simulink subsystem "Simulation_Differential_AGV"  (R2024b)
settings: Solver=VariableStepAuto  StartTime=0.0  StopTime=10.0  RelTol=1e-3
model mask{poseInit=[0 0 0], vInit=[0 0], Ts=0.05, speedLimits=[-2 8]}
  mask prompts: poseInit "Initial position (m,m,rad)"; vInit "Initial speed (m/s, rad/s)"; Ts "Sampling Time (s)"; speedLimits "Speed Limits"
undefined symbols (not defined in the file): DiscIntNeverNeededParam
settings Model: Creator=marti  LastModifiedBy=marti

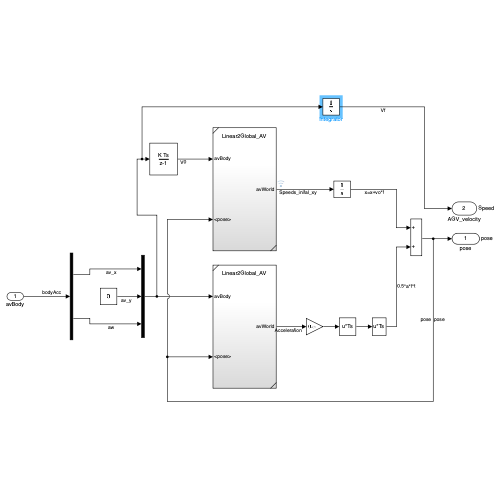
[thumbnail: Simulink's stored preview of the top-level diagram]
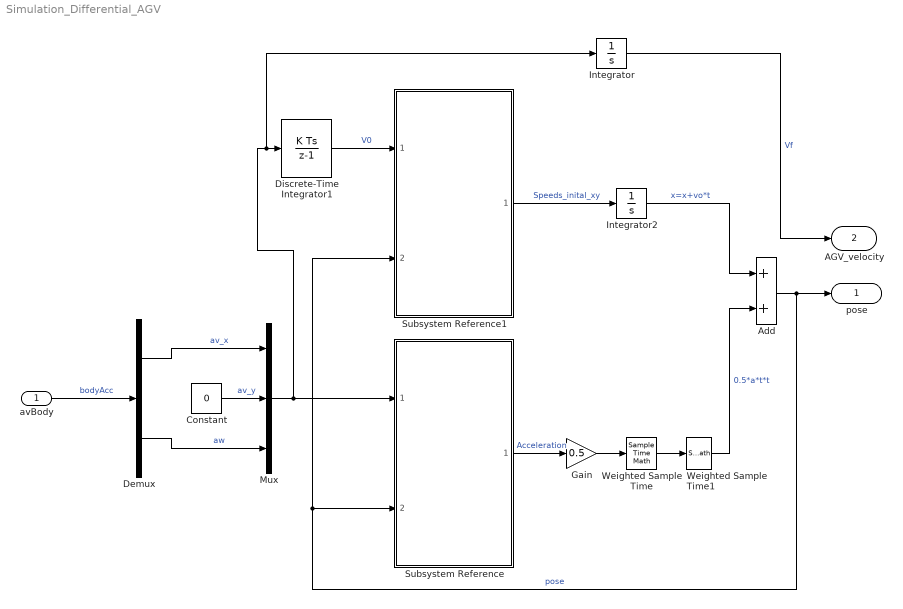
== system Simulation_Differential_AGV ==
  avBody : Inport  PortDimensions=2  SampleTime=Ts
  Add : Sum
  Constant : Constant  Value=0  SampleTime=Ts
  Demux : Demux  Outputs=2
  Discrete-Time Integrator1 : DiscreteIntegrator  InitialCondition=[vInit(1) 0 vInit(2)]  SampleTime=Ts  ICPrevOutput=DiscIntNeverNeededParam  ICPrevScaledInput=DiscIntNeverNeededParam
  Gain : Gain  Gain=0.5
  Integrator : Integrator
  Integrator2 : Integrator  InitialCondition=poseInit
  Mux : Mux  Inputs=3
  Subsystem Reference : Subsystem  ReferencedSubsystem=Linear2Global_AV
  Subsystem Reference1 : Subsystem  ReferencedSubsystem=Linear2Global_AV
  Weighted Sample Time : SampleTimeMath  TsampMathOp=*  weightValue=1
  Weighted Sample Time1 : SampleTimeMath  TsampMathOp=*  weightValue=1
  pose : Outport  SignalName=pose  PortDimensions=3  SampleTime=Ts
  AGV_velocity : Outport  Port=2  SignalName=Speed  SampleTime=Ts
  wires:
  avBody/1 -> Demux/1  "bodyAcc"
  Subsystem Reference/1 -> Gain/1  "Acceleration"
  Weighted Sample Time/1 -> Weighted Sample Time1/1
  Gain/1 -> Weighted Sample Time/1
  Weighted Sample Time1/1 -> Add/2  "0.5*a*t*t"
  Integrator2/1 -> Add/1  "x=x+vo*t"
  Add/1 -> pose/1, Subsystem Reference1/2, Subsystem Reference/2  "pose"
  Constant/1 -> Mux/2  "av_y"
  Demux/1 -> Mux/1  "av_x"
  Demux/2 -> Mux/3  "aw"
  Discrete-Time Integrator1/1 -> Subsystem Reference1/1  "V0"
  Subsystem Reference1/1 -> Integrator2/1  "Speeds_inital_xy"
  Integrator/1 -> AGV_velocity/1  "Vf"
  Mux/1 -> Subsystem Reference/1, Integrator/1, Discrete-Time Integrator1/1
